simulink model "shower_control"  (R2025a)
settings: Solver=VariableStepAuto  StartTime=0.0  StopTime=10.0  RelTol=1e-3
settings Model: Creator=lukelo_g  LastModifiedBy=lukelo_g

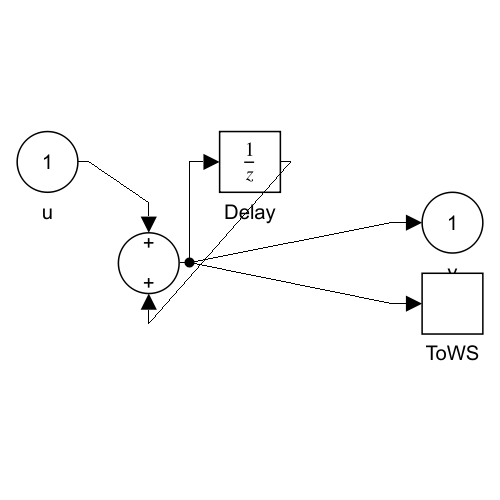
[thumbnail: Simulink's stored preview of the top-level diagram]
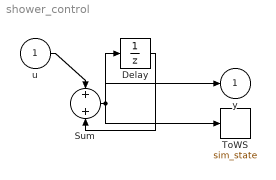
== system shower_control ==
  u : Inport
  Delay : UnitDelay  InitialCondition=36  SampleTime=-1  HasFrameUpgradeWarning=on
  Sum : Sum
  ToWS : ToWorkspace  VariableName=sim_state  SampleTime=-1
  y : Outport
  wires:
  u/1 -> Sum/1
  Delay/1 -> Sum/2
  Sum/1 -> Delay/1, y/1, ToWS/1
